simulink model "q_aero2_2dof_pid_control_test"  (R2021a)
settings: Solver=ode3  StartTime=0.0  StopTime=inf  FixedStep=0.002  RelTol=1e-3  EnableMultiTasking=on
undefined symbols (not defined in the file): HIL, qc_get_step_size
libraries: quarc_library x5, simulink_extras x4
settings Model: ExtModeTrigDuration=10000  Creator=Derek  LastModifiedBy=Derek
settings SolverCC: AlgebraicLoopSolver=TrustRegion  PositivePriorityOrder=on
settings DataIOCC: ReturnWorkspaceOutputs=off
settings DebuggingCC: SFMachineParentedDataDiag=warning  ArithmeticOperatorsInVariantConditions=warning
settings SFSimCC: SimUseLocalCustomCode=off  CustomCodeUndefinedFunction=UseInterfaceOnly
settings RTWCC: Description=QUARC Win64 Target Using Toolchain  SystemTargetFile=quarc_win64.tlc  TemplateMakefile=quarc_default_tmf  RTWUseLocalCustomCode=off  Toolchain=QUARC win64 | nmake (64-bit Windows)  BuildConfiguration=Faster Runs
settings CodeAppCC: StateflowObjectComments=on
settings STFCustomTargetCC: TargetLangStandard=C99 (ISO)  ConcurrentExecutionCompliant=on  SystemTargetFile=quarc_win64.tlc
settings GRTTargetCC: ParMdlRefBuildCompliant=off  CompOptLevelCompliant=off  CombineOutputUpdateFcns=off  MatFileLogging=off  CPPClassGenCompliant=off  GRTInterface=on  ExtMode=on  ExtModeMexFile=quarc_comm
settings ConfigComp: CovMetricSettings=dswe

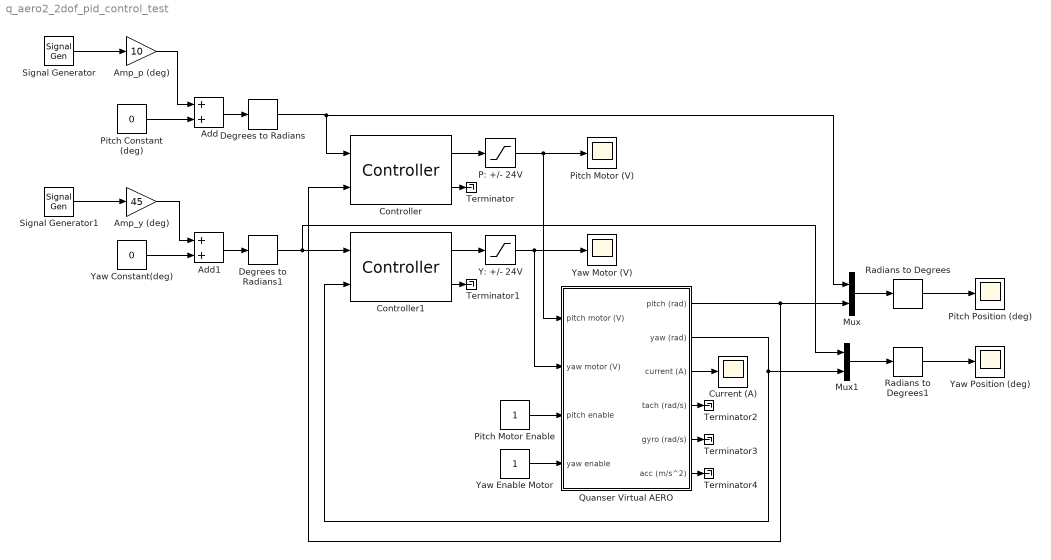
== system q_aero2_2dof_pid_control_test ==
  Add : Sum
  Add1 : Sum
  Amp_p (deg) : Gain  Gain=10
  Amp_y (deg) : Gain  Gain=45
  Controller : quarc_library/Continuous/Controller  ctrl_type=Proportional-Integral-Velocity (PIV)  param_src=Specify via dialog  Kp=107.7  Ki=0  Kd=0  Kv=52.4  Ka=0  Wn=100
      settings: SourceProductName=QUARC Targets
  Controller1 : quarc_library/Continuous/Controller  ctrl_type=Proportional-Integral-Velocity (PIV)  param_src=Specify via dialog  Kp=54.1  Ki=0  Kd=0  Kv=19.6  Ka=0  Wn=100
      settings: SourceProductName=QUARC Targets
  Current (A) : Scope
  Degrees to Radians : simulink_extras/Transformations/Degrees to Radians
  Degrees to Radians1 : simulink_extras/Transformations/Degrees to Radians
  Mux : Mux  Inputs=2
  Mux1 : Mux  Inputs=2
  P: +/- 24V : Saturate  UpperLimit=24  LowerLimit=-24
  Pitch Constant (deg) : Constant  Value=0
  Pitch Motor (V) : Scope
  Pitch Motor Enable : Constant
  Pitch Position (deg) : Scope
  Quanser Virtual AERO : Subsystem
  Radians to Degrees : simulink_extras/Transformations/Radians to Degrees
  Radians to Degrees1 : simulink_extras/Transformations/Radians to Degrees
  Signal Generator : SignalGenerator  WaveForm=square  Frequency=0.1
  Signal Generator1 : SignalGenerator  WaveForm=square  Frequency=0.04
  Terminator{,1..4} (5 alike) : Terminator
  Y: +/- 24V : Saturate  UpperLimit=24  LowerLimit=-24
  Yaw Constant(deg) : Constant  Value=0
  Yaw Enable Motor : Constant
  Yaw Motor (V) : Scope
  Yaw Position (deg) : Scope
  wires:
  P: +/- 24V/1 -> Quanser Virtual AERO/1(pitch motor (V)), Pitch Motor (V)/1
  Yaw Enable Motor/1 -> Quanser Virtual AERO/4(yaw enable)
  Mux/1 -> Radians to Degrees/1
  Quanser Virtual AERO/6(acc (m/s^2)) -> Terminator4/1
  Y: +/- 24V/1 -> Quanser Virtual AERO/2(yaw motor (V)), Yaw Motor (V)/1
  Pitch Motor Enable/1 -> Quanser Virtual AERO/3(pitch enable)
  Quanser Virtual AERO/5(gyro (rad/s)) -> Terminator3/1
  Radians to Degrees1/1 -> Yaw Position (deg)/1
  Controller/2 -> Terminator/1
  Quanser Virtual AERO/4(tach (rad/s)) -> Terminator2/1
  Controller/1 -> P: +/- 24V/1
  Mux1/1 -> Radians to Degrees1/1
  Degrees to Radians1/1 -> Controller1/1, Mux1/1
  Signal Generator1/1 -> Amp_y (deg)/1
  Quanser Virtual AERO/2(yaw (rad)) -> Controller1/2, Mux1/2
  Controller1/1 -> Y: +/- 24V/1
  Add1/1 -> Degrees to Radians1/1
  Yaw Constant(deg)/1 -> Add1/2
  Add/1 -> Degrees to Radians/1
  Pitch Constant (deg)/1 -> Add/2
  Signal Generator/1 -> Amp_p (deg)/1
  Controller1/2 -> Terminator1/1
  Quanser Virtual AERO/1(pitch (rad)) -> Controller/2, Mux/2
  Radians to Degrees/1 -> Pitch Position (deg)/1
  Amp_y (deg)/1 -> Add1/1
  Amp_p (deg)/1 -> Add/1
  Quanser Virtual AERO/3(current (A)) -> Current (A)/1
  Degrees to Radians/1 -> Mux/1, Controller/1

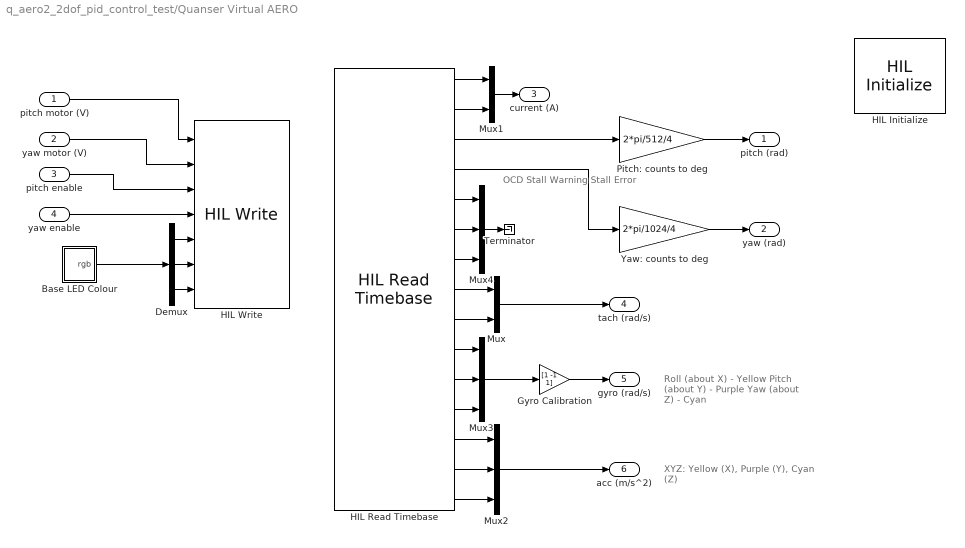
== system q_aero2_2dof_pid_control_test/Quanser Virtual AERO ==
  note: OCD
      | Stall Warning
      | Stall Error
  note: XYZ:
      | Yellow (X), Purple (Y), Cyan (Z)
  note: Roll (about X) - Yellow
      | Pitch (about Y) - Purple
      | Yaw (about Z) - Cyan
  pitch motor (V) : Inport
  yaw motor (V) : Inport  Port=2
  pitch enable : Inport  Port=3
  yaw enable : Inport  Port=4
  Base LED Colour : Subsystem  mask(Color Constant){color=[0 1 0]}
      mask help: Outputs a constant RGB color value.
      mask init:
      | rgb = get_param(gcbh, 'color');
      | if numel(color) ~= 3
      |     rgb = [0 0 0];
      | end
      | set_param(gcbh, 'MaskDisplay', ['patch([-0.02 -0.02 1.02 1.02], [-0.02 1.02 1.02 -0.02], ', rgb, ');']);
      settings: OpenFcn=color_constant_properties('CurrentBlock', gcbh);
      mask Help: web(qc_get_block_help_path(gcb), '-helpbrowser');
      mask Display: patch([-0.02 -0.02 1.02 1.02], [-0.02 1.02 1.02 -0.02], [0 1 0]);
  Demux : Demux  Outputs=3
  Gyro Calibration : Gain  Gain=[1 -1 1]
  HIL Initialize : quarc_library/Data Acquisition/Generic/Configuration/HIL Initialize  Priority=-99  object_name=HIL-1  board_type=quanser_aero2_usb  board_number=0@tcpip://localhost:18930  board_options=""  exclusive=off  active=on  hardware_clocks=[0]  clock_modes=[]  initial_clock_frequencies=[]  set_clock_params_at_start=off  set_clock_params_at_switch_in=off  set_clock_frequencies_at_start=off  set_clock_frequencies_at_switch_in=off  analog_input_channels=[0:1]  analog_input_configurations=[]  analog_input_maximums=3  analog_input_minimums=-3  set_analog_input_params_at_start=off  set_analog_input_params_at_switch_in=off  analog_output_channels=[0:1]  analog_output_maximums=24  analog_output_minimums=-24  initial_analog_outputs=[0]  final_analog_outputs=[0]  watchdog_analog_outputs=[0]  set_analog_output_params_at_start=off  set_analog_output_params_at_switch_in=off  set_analog_outputs_at_start=on  set_analog_outputs_at_switch_in=off  set_analog_outputs_at_terminate=on  set_analog_outputs_at_switch_out=off  set_analog_outputs_on_watchdog=on  digital_input_channels=[]  digital_output_channels=[0:1]  digital_output_configuration=[]  initial_digital_outputs=[1]  final_digital_outputs=[0]  watchdog_digital_outputs=[0]  set_digital_output_params_at_start=off  set_digital_output_params_at_switch_in=off  set_digital_outputs_at_start=on  set_digital_outputs_at_switch_in=off  set_digital_outputs_at_terminate=on  set_digital_outputs_at_switch_out=off  set_digital_outputs_on_watchdog=on  encoder_channels=[0:3]  quadrature=[4]  encoder_filter_frequency=[]  initial_encoder_counts=[0]  set_encoder_params_at_start=off  set_encoder_params_at_switch_in=off  set_encoder_counts_at_start=on  set_encoder_counts_at_switch_in=off  pwm_channels=[]  pwm_modes=[]  pwm_frequency=[]  pwm_configuration=[]  pwm_alignment=[]  pwm_polarity=[]  pwm_leading_deadband=[]  pwm_trailing_deadband=[]  initial_pwm_outputs=[]  final_pwm_outputs=[]  watchdog_pwm_outputs=[]  set_pwm_params_at_start=off  set_pwm_params_at_switch_in=off  set_pwm_outputs_at_start=off  set_pwm_outputs_at_switch_in=off  set_pwm_outputs_at_terminate=off  set_pwm_outputs_at_switch_out=off  set_pwm_outputs_on_watchdog=off  other_output_channels=[11000:11002]  initial_other_outputs=[0 1 0]  final_other_outputs=[1 0 0]  watchdog_other_outputs=[0 0 1]  set_other_outputs_at_start=on  set_other_outputs_at_switch_in=off  set_other_outputs_at_terminate=on  set_other_outputs_at_switch_out=off  set_other_outputs_on_watchdog=on
  HIL Read Timebase : quarc_library/Data Acquisition/Generic/Timebases/HIL Read Timebase  object_name=HIL-1  clock=0  analog_channels=[0:1]  encoder_channels=[2:3]  digital_channels=[0:2]  other_channels=[14000:14001 3000:3002 4000:4002]  active=on  vector_output=off  data_type_mode=Inherit via back propagation  encoder_data_type=double  digital_data_type=boolean  overflow_mode=Synchronize (for simulated cards only)  samples_in_buffer=1+0*max(ceil(1/qc_get_step_size), 1)
  HIL Write : quarc_library/Data Acquisition/Generic/Immediate I//O/HIL Write  object_name=HIL-1  analog_channels=[0:1]  pwm_channels=[]  digital_channels=[0:1]  other_channels=[11000:11002]  sample_time=-1  active=on  vector_input=off
  Mux : Mux  Inputs=2
  Mux1 : Mux  Inputs=2
  Mux2 : Mux  Inputs=3
  Mux3 : Mux  Inputs=3
  Mux4 : Mux  Inputs=3
  Pitch: counts to deg : Gain  Gain=2*pi/512/4
  Terminator : Terminator
  Yaw: counts to deg : Gain  Gain=2*pi/1024/4
  pitch (rad) : Outport  VectorParamsAs1DForOutWhenUnconnected=off
  yaw (rad) : Outport  Port=2  VectorParamsAs1DForOutWhenUnconnected=off
  current (A) : Outport  Port=3  VectorParamsAs1DForOutWhenUnconnected=off
  tach (rad/s) : Outport  Port=4  VectorParamsAs1DForOutWhenUnconnected=off
  gyro (rad/s) : Outport  Port=5  VectorParamsAs1DForOutWhenUnconnected=off
  acc (m/s^2) : Outport  Port=6  VectorParamsAs1DForOutWhenUnconnected=off
  wires:
  Mux4/1 -> Terminator/1
  HIL Read Timebase/7 -> Mux4/3
  HIL Read Timebase/6 -> Mux4/2
  HIL Read Timebase/5 -> Mux4/1
  HIL Read Timebase/9 -> Mux/2
  HIL Read Timebase/8 -> Mux/1
  HIL Read Timebase/12 -> Mux3/3
  HIL Read Timebase/11 -> Mux3/2
  HIL Read Timebase/10 -> Mux3/1
  HIL Read Timebase/13 -> Mux2/1
  HIL Read Timebase/14 -> Mux2/2
  HIL Read Timebase/15 -> Mux2/3
  Mux/1 -> tach (rad/s)/1
  yaw motor (V)/1 -> HIL Write/2
  Gyro Calibration/1 -> gyro (rad/s)/1
  Mux3/1 -> Gyro Calibration/1
  HIL Read Timebase/4 -> Yaw: counts to deg/1
  HIL Read Timebase/3 -> Pitch: counts to deg/1
  Mux1/1 -> current (A)/1
  pitch motor (V)/1 -> HIL Write/1
  Pitch: counts to deg/1 -> pitch (rad)/1
  Yaw: counts to deg/1 -> yaw (rad)/1
  HIL Read Timebase/2 -> Mux1/2
  HIL Read Timebase/1 -> Mux1/1
  Demux/3 -> HIL Write/7
  Demux/2 -> HIL Write/6
  Demux/1 -> HIL Write/5
  Base LED Colour/1(rgb) -> Demux/1
  yaw enable/1 -> HIL Write/4
  pitch enable/1 -> HIL Write/3
  Mux2/1 -> acc (m/s^2)/1

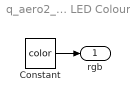
== system q_aero2_2dof_pid_control_test/Quanser Virtual AERO/Base LED Colour ==
  Constant : Constant  Value=color
  rgb : Outport  VectorParamsAs1DForOutWhenUnconnected=off
  wires:
  Constant/1 -> rgb/1
